simulink model "lab2_part2"  (R2022a)
settings: Solver=VariableStepAuto  StartTime=0.0  StopTime=30.0  RelTol=1e-10  AbsTol=1e-10
values from neighbouring files (symbols this model uses):
  A = [0 1; 0 -alpha_2/M]    [lab2.m]
  Actrl = A + B*K - L*C    [lab2.m]
  B = [0; alpha_1/M]    [lab2.m]
  Bctrl = [L -B*K]    [lab2.m]
  C = [1 0]    [lab2.m]
  Cctrl = K    [lab2.m]
  Dctrl = [0 -K]    [lab2.m]
settings Model: Creator=dell  LastModifiedBy=jiaoaora
settings ModelReferenceCC: EnableRefExpFcnMdlSchedulingChecks=off
settings RTWCC: Description=Generic Real-Time Target

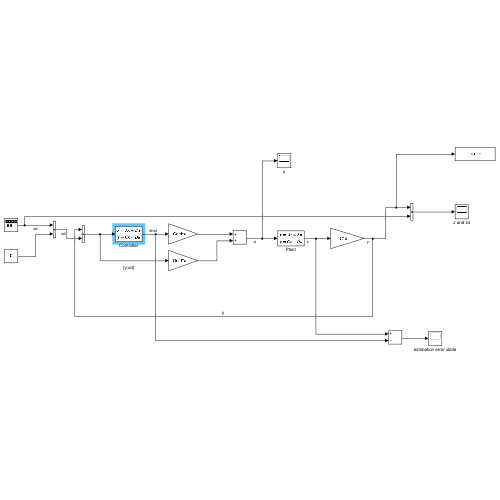
[thumbnail: Simulink's stored preview of the top-level diagram]
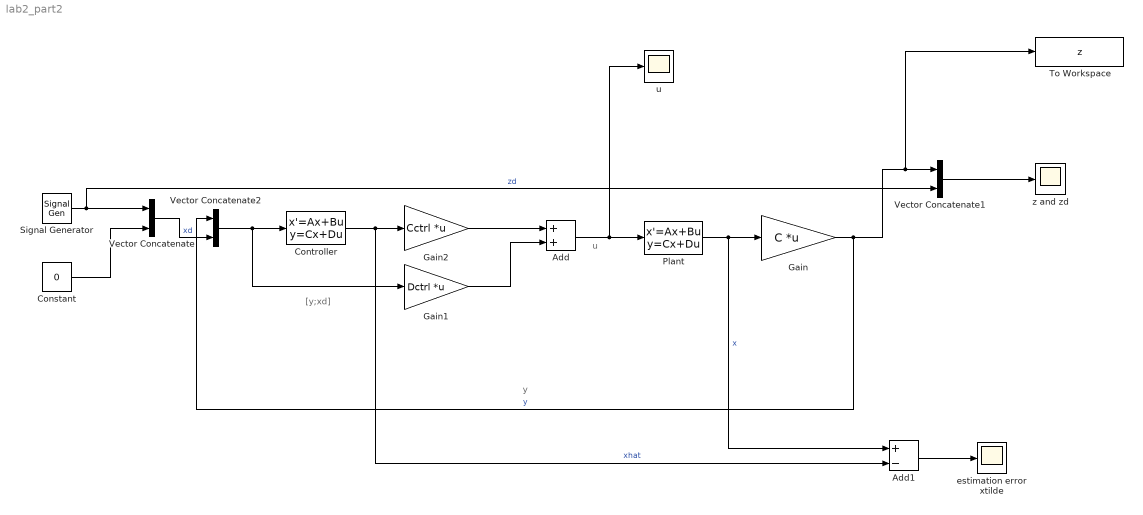
== system lab2_part2 ==
  note: [y;xd]
  note: u
  note: y
  Add : Sum
  Add1 : Sum  Inputs=+-
  Constant : Constant  Value=0
  Controller : StateSpace  A=Actrl  B=Bctrl  C=eye(2)  D=zeros(2, 3)  InitialCondition=1
  Gain : Gain  Gain=C  Multiplication=Matrix(K*u)
  Gain1 : Gain  Gain=Dctrl  Multiplication=Matrix(K*u)
  Gain2 : Gain  Gain=Cctrl  Multiplication=Matrix(K*u)
  Plant : StateSpace  A=A  B=B  C=eye(2)  D=zeros(2, 1)  InitialCondition=0  ParameterTunability=Unconstrained
  Signal Generator : SignalGenerator  WaveForm=square  Amplitude=0.03  Frequency=0.1
  To Workspace : ToWorkspace  VariableName=z  SaveFormat=Timeseries  SampleTime=-1
  Vector Concatenate : Concatenate
  Vector Concatenate1 : Concatenate
  Vector Concatenate2 : Concatenate
  estimation error xtilde : Scope
  u : Scope
  z and zd : Scope
  wires:
  Vector Concatenate1/1 -> z and zd/1
  Plant/1 -> Add1/1, Gain/1  "x"
  Constant/1 -> Vector Concatenate/2
  Signal Generator/1 -> Vector Concatenate1/2, Vector Concatenate/1  "zd"
  Vector Concatenate/1 -> Vector Concatenate2/2  "xd"
  Vector Concatenate2/1 -> Gain1/1, Controller/1
  Controller/1 -> Add1/2, Gain2/1  "xhat"
  Add/1 -> u/1, Plant/1
  Gain/1 -> Vector Concatenate2/1, To Workspace/1, Vector Concatenate1/1  "y"
  Gain1/1 -> Add/2
  Add1/1 -> estimation error xtilde/1
  Gain2/1 -> Add/1
